simulink model "sf_pw_switch3_"  (Simulink 7.4)
settings: Solver=ode45  StartTime=0.0  StopTime=10.0  RelTol=1e-3
settings Model: Creator=rcobbe  LastModifiedBy=rcobbe

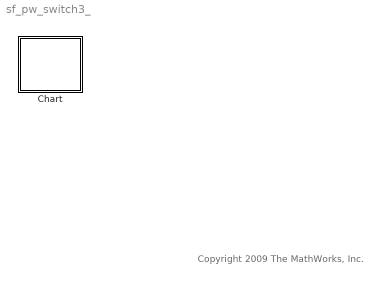
== system sf_pw_switch3_ ==
  note: Copyright 2009 The MathWorks, Inc.
  Chart : Stateflow chart

== stateflow chart Chart ==
  note: Do not put any code along
      | the transitions that run
      | down the right side!
  (junction 12) -> (junction 4) [order 1] : [case1]
  (junction 4) -> (junction 5) : {action1}
  (junction 5) -> (junction 13)
  (junction 13) -> (junction 9)
  (junction 14) -> (junction 7) [order 1] : [case2]
  (junction 7) -> (junction 6) : {action2}
  (junction 6) -> (junction 9)
  (junction 12) -> (junction 14) [order 2]
  (junction 14) -> (junction 15) [order 2]
  (junction 9) -> (junction 8)
  (junction 15) -> (junction 10) [order 1] : [case3]
  (junction 10) -> (junction 11) : {action3}
  (junction 11) -> (junction 8)
  (junction 8) -> (junction 16)
  (junction 15) -> (junction 17) [order 2] : {defaultAction}
  (default) -> (junction 12) : /*comment*/
  (junction 16) -> (junction 17)
  (junction 17) -> (junction 18)
